simulink model "HaFu1"  (Simulink 7.1)
settings: Solver=ode45  StartTime=0.0  StopTime=1000.0  RelTol=1e-3
settings Model: Creator=Meisel  LastModifiedBy=Meisel

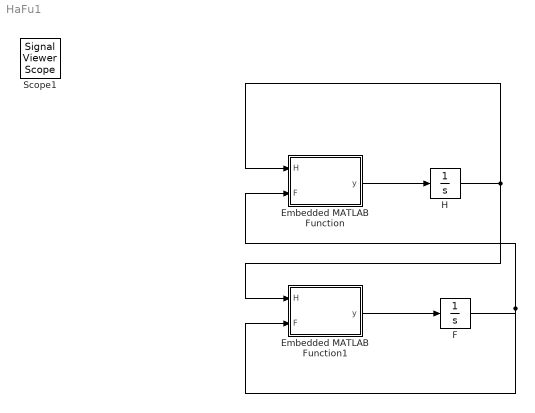
== system HaFu1 ==
  Embedded MATLAB Function : Stateflow chart
  Embedded MATLAB Function1 : Stateflow chart
  F : Integrator  InitialCondition=50
  H : Integrator  InitialCondition=200
  Scope1 : SignalViewerScope  IOType=viewer  RefreshTime=0.035000
      settings: TimeRange=1000  YMin=20  YMax=220
  wires:
  Embedded MATLAB Function/1(y) -> H/1
  H/1 -> Embedded MATLAB Function/1(H), Embedded MATLAB Function1/1(H)
  F/1 -> Embedded MATLAB Function/2(F), Embedded MATLAB Function1/2(F)
  Embedded MATLAB Function1/1(y) -> F/1

== matlab function Embedded MATLAB Function1 ==
  data: H input double; y output double; F input double
function y = fcn(H, F)
% This block supports the Embedded MATLAB subset.
% See the help menu for details. 

y = -0.01*F + 0.0001*H*F - 0.000000001*F*F;

== matlab function Embedded MATLAB Function ==
  data: H input double; y output double; F input double
function y = fcn(H, F)
% This block supports the Embedded MATLAB subset.
% See the help menu for details. 

y = 0.02*H - 0.0005*H*F - 0.00000001*H*H;
